simulink model "MHILSimHWImpl"  (R2024a)
settings: Solver=FixedStepDiscrete  StartTime=0.0  StopTime=2e-4  FixedStep=4e-9  RelTol=1e-3
values from neighbouring files (symbols this model uses):
  cfg = tddbl_model    [HILSimModel.m]
undefined symbols (not defined in the file or in its folder): AXI4, dt, hw, ip, Lite, xc7z020clg400
libraries: hdlBasic x1497, hdlUtilities x3, vmcUtilities x1
(part 8 of 11)

== system MHILSimHWImpl/hilsim_ipcore/proc_domain/slice_1/int_xddot_xdot ==
  ts_sync_in : Inport
  reset_in : Inport  Port=2
  xdot : Inport  Port=3
  Constant : hdlBasic/Constant  const=ip.int_dt_residual  gui_display_data_type=Fixed-point  arith_type=Signed (2's comp)  n_bits=dt.const.sz  bin_pt=dt.const.bin  preci_type=Single  exp_width=8  frac_width=24  explicit_period=off  period=1  XmcBlockStatus=1  maskContainerNames=tabcontainer1  block_type=constant  block_config=sysgen:Constant_config
  Register : hdlBasic/Register  init=0  rst=on  en=on  XmcBlockStatus=1  maskContainerNames=tabcontainer1  block_type=register  block_config=sysgen:Register_config
  Register1 : hdlBasic/Register  init=0  rst=on  en=on  XmcBlockStatus=1  maskContainerNames=tabcontainer1  block_type=register  block_config=sysgen:Register_config
  add_stage_1 : hdlBasic/AddSub  mode=Addition  use_carryin=off  use_carryout=off  en=off  latency=1  precision=User Defined  arith_type="Signed  (2's comp)"  n_bits=dt.slice.sz  bin_pt=dt.slice.bin  quantization=Truncate  overflow=Wrap  use_behavioral_HDL=off  hw_selection=Fabric  pipelined=off  XmcBlockStatus=1  maskContainerNames=tabcontainer1  block_type=addsub  block_config=sysgen:Addsub_config
  add_stage_2 : hdlBasic/AddSub  mode=Subtraction  use_carryin=off  use_carryout=off  en=off  latency=1  precision=User Defined  arith_type="Signed  (2's comp)"  n_bits=dt.slice.sz  bin_pt=dt.slice.bin  quantization=Truncate  overflow=Wrap  use_behavioral_HDL=off  hw_selection=Fabric  pipelined=off  XmcBlockStatus=1  maskContainerNames=tabcontainer1  block_type=addsub  block_config=sysgen:Addsub_config
  deltat_residual_mult : hdlBasic/Mult  precision=User Defined  arith_type="Signed  (2's comp)"  n_bits=dt.slice.sz  bin_pt=dt.slice.bin  quantization=Truncate  overflow=Wrap  en=off  latency=2  opt_float=off  fp_mult_usage=No Usage  use_behavioral_HDL=off  opt=Speed  use_embedded=on  optimum_pipeline=off  pipeline=on  use_rpm=on  placement_style=Triangular  XmcBlockStatus=1  maskContainerNames=group1  block_type=mult  block_config=sysgen:Mult_config  block_width=598  block_height=876
  half : hdlBasic/Scale  scale_factor=-1  XmcBlockStatus=1  maskContainerNames=group1  block_type=scale  block_config=sysgen:Scale_config
  int_accum : hdlBasic/AddSub  mode=Addition  use_carryin=off  use_carryout=off  en=off  latency=2  precision=User Defined  arith_type="Signed  (2's comp)"  n_bits=dt.accum.sz  bin_pt=dt.accum.bin  quantization=Truncate  overflow=Saturate  use_behavioral_HDL=off  hw_selection=DSP48  pipelined=on  XmcBlockStatus=1  maskContainerNames=tabcontainer1  block_type=addsub  block_config=sysgen:Addsub_config
  prepend_zeros : hdlBasic/Convert  gui_display_data_type=Fixed-point  arith_type=Signed (2's comp)  n_bits=dt.slice.sz + ip.int_scale_bits  bin_pt=dt.slice.bin  float_type=Single  exp_bits=8  fraction_bits=24  quantization=Truncate  overflow=Wrap  en=off  latency=0  pipeline=off  XmcBlockStatus=1  maskContainerNames=group2  block_type=convert  block_config=sysgen:Convert_config  block_width=595  block_height=885
  shift_prescale : hdlBasic/Scale  scale_factor=-ip.int_scale_bits  XmcBlockStatus=1  maskContainerNames=group1  block_type=scale  block_config=sysgen:Scale_config
  x : Outport
  wires:
  shift_prescale/1 -> int_accum/1
  prepend_zeros/1 -> shift_prescale/1
  Constant/1 -> deltat_residual_mult/2
  deltat_residual_mult/1 -> prepend_zeros/1
  ts_sync_in/1 -> Register/3, Register1/3
  int_accum/1 -> x/1, Register/1
  add_stage_1/1 -> add_stage_2/1
  half/1 -> Register1/1, add_stage_1/2
  reset_in/1 -> Register/2, Register1/2
  Register/1 -> int_accum/2
  Register1/1 -> add_stage_2/2
  xdot/1 -> add_stage_1/1, half/1
  add_stage_2/1 -> deltat_residual_mult/1

== system MHILSimHWImpl/hilsim_ipcore/proc_domain/slice_1/int_xdot_x ==
  ts_sync_in : Inport
  reset_in : Inport  Port=2
  xdot : Inport  Port=3
  Constant : hdlBasic/Constant  const=ip.int_dt_residual  gui_display_data_type=Fixed-point  arith_type=Signed (2's comp)  n_bits=dt.const.sz  bin_pt=dt.const.bin  preci_type=Single  exp_width=8  frac_width=24  explicit_period=off  period=1  XmcBlockStatus=1  maskContainerNames=tabcontainer1  block_type=constant  block_config=sysgen:Constant_config
  Register : hdlBasic/Register  init=0  rst=on  en=on  XmcBlockStatus=1  maskContainerNames=tabcontainer1  block_type=register  block_config=sysgen:Register_config
  Register1 : hdlBasic/Register  init=0  rst=on  en=on  XmcBlockStatus=1  maskContainerNames=tabcontainer1  block_type=register  block_config=sysgen:Register_config
  add_stage_3 : hdlBasic/AddSub  mode=Addition  use_carryin=off  use_carryout=off  en=off  latency=1  precision=User Defined  arith_type="Signed  (2's comp)"  n_bits=dt.slice.sz  bin_pt=dt.slice.bin  quantization=Truncate  overflow=Wrap  use_behavioral_HDL=off  hw_selection=Fabric  pipelined=off  XmcBlockStatus=1  maskContainerNames=tabcontainer1  block_type=addsub  block_config=sysgen:Addsub_config
  deltat_residual_mult : hdlBasic/Mult  precision=User Defined  arith_type="Signed  (2's comp)"  n_bits=dt.slice.sz  bin_pt=dt.slice.bin  quantization=Truncate  overflow=Wrap  en=off  latency=2  opt_float=off  fp_mult_usage=No Usage  use_behavioral_HDL=off  opt=Speed  use_embedded=on  optimum_pipeline=off  pipeline=on  use_rpm=on  placement_style=Triangular  XmcBlockStatus=1  maskContainerNames=group1  block_type=mult  block_config=sysgen:Mult_config  block_width=598  block_height=876
  half1 : hdlBasic/Scale  scale_factor=-1  XmcBlockStatus=1  maskContainerNames=group1  block_type=scale  block_config=sysgen:Scale_config
  int_accum : hdlBasic/AddSub  mode=Addition  use_carryin=off  use_carryout=off  en=off  latency=2  precision=User Defined  arith_type="Signed  (2's comp)"  n_bits=dt.accum.sz  bin_pt=dt.accum.bin  quantization=Truncate  overflow=Saturate  use_behavioral_HDL=off  hw_selection=DSP48  pipelined=on  XmcBlockStatus=1  maskContainerNames=tabcontainer1  block_type=addsub  block_config=sysgen:Addsub_config
  prepend_zeros : hdlBasic/Convert  gui_display_data_type=Fixed-point  arith_type="Signed  (2's comp)"  n_bits=dt.slice.sz + ip.int_scale_bits  bin_pt=dt.slice.bin  float_type=Single  exp_bits=8  fraction_bits=24  quantization=Truncate  overflow=Wrap  en=off  latency=0  pipeline=off  XmcBlockStatus=1  maskContainerNames=group2  block_type=convert  block_config=sysgen:Convert_config  block_width=595  block_height=885
  shift_prescale : hdlBasic/Scale  scale_factor=-ip.int_scale_bits  XmcBlockStatus=1  maskContainerNames=group1  block_type=scale  block_config=sysgen:Scale_config
  x : Outport
  wires:
  shift_prescale/1 -> int_accum/1
  prepend_zeros/1 -> shift_prescale/1
  Constant/1 -> deltat_residual_mult/2
  deltat_residual_mult/1 -> prepend_zeros/1
  int_accum/1 -> Register/1, x/1
  Register/1 -> int_accum/2
  add_stage_3/1 -> half1/1
  Register1/1 -> add_stage_3/2
  ts_sync_in/1 -> Register1/3, Register/3
  reset_in/1 -> Register1/2, Register/2
  xdot/1 -> Register1/1, add_stage_3/1
  half1/1 -> deltat_residual_mult/1

== system MHILSimHWImpl/hilsim_ipcore/proc_domain/slice_1/x_psc ==
  in : Inport
  presc_shift : Inport  Port=2
  presc_mul : Inport  Port=3
  barrel_left_shifter : Subsystem
  cast_to_dt/slice : hdlBasic/Convert  gui_display_data_type=Fixed-point  arith_type="Signed  (2's comp)"  n_bits=dt.slice.sz  bin_pt=dt.slice.bin  float_type=Single  exp_bits=8  fraction_bits=24  quantization=Truncate  overflow=Wrap  en=off  latency=0  pipeline=off  XmcBlockStatus=1  maskContainerNames=group2  block_type=convert  block_config=sysgen:Convert_config  block_width=595  block_height=885
  mult_presc : hdlBasic/Mult  precision=User Defined  arith_type="Signed  (2's comp)"  n_bits=dt.slice.sz  bin_pt=dt.slice.bin  quantization=Truncate  overflow=Wrap  en=off  latency=2  opt_float=off  fp_mult_usage=No Usage  use_behavioral_HDL=off  opt=Speed  use_embedded=on  optimum_pipeline=off  pipeline=on  use_rpm=on  placement_style=Triangular  XmcBlockStatus=1  maskContainerNames=group1  block_type=mult  block_config=sysgen:Mult_config  block_width=598  block_height=876
  out : Outport
  wires:
  presc_mul/1 -> mult_presc/2
  barrel_left_shifter/1(out) -> cast_to_dt/slice/1
  cast_to_dt/slice/1 -> mult_presc/1
  mult_presc/1 -> out/1
  presc_shift/1 -> barrel_left_shifter/2(shift_by)
  in/1 -> barrel_left_shifter/1(in)

== system MHILSimHWImpl/hilsim_ipcore/proc_domain/slice_1/xdot_psc ==
  in : Inport
  presc_shift : Inport  Port=2
  presc_mul : Inport  Port=3
  barrel_left_shifter : Subsystem
  cast_to_dt/slice : hdlBasic/Convert  gui_display_data_type=Fixed-point  arith_type=Signed (2's comp)  n_bits=dt.slice.sz  bin_pt=dt.slice.bin  float_type=Single  exp_bits=8  fraction_bits=24  quantization=Truncate  overflow=Wrap  en=off  latency=0  pipeline=off  XmcBlockStatus=1  maskContainerNames=group2  block_type=convert  block_config=sysgen:Convert_config  block_width=595  block_height=885
  mult_presc : hdlBasic/Mult  precision=User Defined  arith_type="Signed  (2's comp)"  n_bits=dt.slice.sz  bin_pt=dt.slice.bin  quantization=Truncate  overflow=Wrap  en=off  latency=2  opt_float=off  fp_mult_usage=No Usage  use_behavioral_HDL=off  opt=Speed  use_embedded=on  optimum_pipeline=off  pipeline=on  use_rpm=on  placement_style=Triangular  XmcBlockStatus=1  maskContainerNames=group1  block_type=mult  block_config=sysgen:Mult_config  block_width=598  block_height=876
  out : Outport
  wires:
  presc_mul/1 -> mult_presc/2
  barrel_left_shifter/1(out) -> cast_to_dt/slice/1
  cast_to_dt/slice/1 -> mult_presc/1
  mult_presc/1 -> out/1
  presc_shift/1 -> barrel_left_shifter/2(shift_by)
  in/1 -> barrel_left_shifter/1(in)

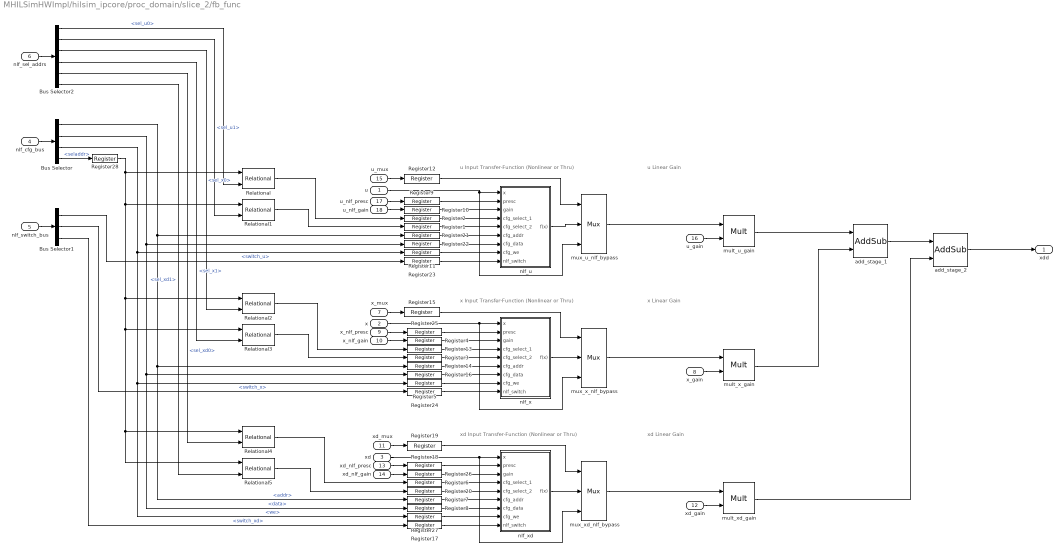
== system MHILSimHWImpl/hilsim_ipcore/proc_domain/slice_2/fb_func ==
  note: u Linear Gain
  note: x Linear Gain
  note: xd Linear Gain
  note: x Input Transfer-Function (Nonlinear or Thru)
  note: xd Input Transfer-Function (Nonlinear or Thru)
  note: u Input Transfer-Function (Nonlinear or Thru)
  u : Inport
  x : Inport  Port=2
  xd : Inport  Port=3
  nlf_cfg_bus : Inport  Port=4
  nlf_switch_bus : Inport  Port=5
  nlf_sel_addrs : Inport  Port=6
  x_mux : Inport  Port=7
  x_gain : Inport  Port=8
  x_nlf_presc : Inport  Port=9
  x_nlf_gain : Inport  Port=10
  xd_mux : Inport  Port=11
  xd_gain : Inport  Port=12
  xd_nlf_presc : Inport  Port=13
  xd_nlf_gain : Inport  Port=14
  u_mux : Inport  Port=15
  u_gain : Inport  Port=16
  u_nlf_presc : Inport  Port=17
  u_nlf_gain : Inport  Port=18
  Bus Selector : BusSelector  OutputSignals=addr,data,we,seladdr
  Bus Selector1 : BusSelector  OutputSignals=switch_u,switch_x,switch_xd
  Bus Selector2 : BusSelector  OutputSignals=sel_u0,sel_u1,sel_x0,sel_x1,sel_xd0,sel_xd1
  Register{1..28} (28 alike) : hdlBasic/Register  init=0  rst=off  en=off  XmcBlockStatus=1  maskContainerNames=tabcontainer1  block_type=register  block_config=sysgen:Register_config
  Relational{,1..5} (6 alike) : hdlBasic/Relational  mode=a=b  op_type=Bool  en=off  latency=1  XmcBlockStatus=1  maskContainerNames=tabcontainer1  block_type=relational  block_config=sysgen:Relational_config
  add_stage_1 : hdlBasic/AddSub  mode=Addition  use_carryin=off  use_carryout=off  en=off  latency=1  precision=User Defined  arith_type="Signed  (2's comp)"  n_bits=dt.slice.sz  bin_pt=dt.slice.bin  quantization=Truncate  overflow=Wrap  use_behavioral_HDL=off  hw_selection=Fabric  pipelined=off  XmcBlockStatus=1  maskContainerNames=tabcontainer1  block_type=addsub  block_config=sysgen:Addsub_config
  add_stage_2 : hdlBasic/AddSub  mode=Addition  use_carryin=off  use_carryout=off  en=off  latency=1  precision=User Defined  arith_type="Signed  (2's comp)"  n_bits=dt.slice.sz  bin_pt=dt.slice.bin  quantization=Truncate  overflow=Wrap  use_behavioral_HDL=off  hw_selection=Fabric  pipelined=off  XmcBlockStatus=1  maskContainerNames=tabcontainer1  block_type=addsub  block_config=sysgen:Addsub_config
  mult_u_gain : hdlBasic/Mult  precision=User Defined  arith_type="Signed  (2's comp)"  n_bits=dt.slice.sz  bin_pt=dt.slice.bin  quantization=Truncate  overflow=Wrap  en=off  latency=2  opt_float=off  fp_mult_usage=No Usage  use_behavioral_HDL=off  opt=Speed  use_embedded=on  optimum_pipeline=off  pipeline=on  use_rpm=on  placement_style=Triangular  XmcBlockStatus=1  maskContainerNames=group1  block_type=mult  block_config=sysgen:Mult_config  block_width=598  block_height=876
  mult_x_gain : hdlBasic/Mult  precision=User Defined  arith_type="Signed  (2's comp)"  n_bits=dt.slice.sz  bin_pt=dt.slice.bin  quantization=Truncate  overflow=Wrap  en=off  latency=2  opt_float=off  fp_mult_usage=No Usage  use_behavioral_HDL=off  opt=Speed  use_embedded=on  optimum_pipeline=off  pipeline=on  use_rpm=on  placement_style=Triangular  XmcBlockStatus=1  maskContainerNames=group1  block_type=mult  block_config=sysgen:Mult_config  block_width=598  block_height=876
  mult_xd_gain : hdlBasic/Mult  precision=User Defined  arith_type="Signed  (2's comp)"  n_bits=dt.slice.sz  bin_pt=dt.slice.bin  quantization=Truncate  overflow=Wrap  en=off  latency=2  opt_float=off  fp_mult_usage=No Usage  use_behavioral_HDL=off  opt=Speed  use_embedded=on  optimum_pipeline=off  pipeline=on  use_rpm=on  placement_style=Triangular  XmcBlockStatus=1  maskContainerNames=group1  block_type=mult  block_config=sysgen:Mult_config  block_width=598  block_height=876
  mux_u_nlf_bypass : hdlBasic/Mux  inputs=2  en=off  latency=1  precision=Full  arith_type=Unsigned  n_bits=16  bin_pt=14  quantization=Truncate  overflow=Wrap  XmcBlockStatus=1  maskContainerNames=tabcontainer1  block_type=mux  block_config=sysgen:Mux_config
  mux_x_nlf_bypass : hdlBasic/Mux  inputs=2  en=off  latency=1  precision=Full  arith_type=Unsigned  n_bits=16  bin_pt=14  quantization=Truncate  overflow=Wrap  XmcBlockStatus=1  maskContainerNames=tabcontainer1  block_type=mux  block_config=sysgen:Mux_config
  mux_xd_nlf_bypass : hdlBasic/Mux  inputs=2  en=off  latency=1  precision=Full  arith_type=Unsigned  n_bits=16  bin_pt=14  quantization=Truncate  overflow=Wrap  XmcBlockStatus=1  maskContainerNames=tabcontainer1  block_type=mux  block_config=sysgen:Mux_config
  nlf_u : Subsystem
  nlf_x : Subsystem
  nlf_xd : Subsystem
  xdd : Outport
  wires:
  x_gain/1 -> mult_x_gain/2
  mux_x_nlf_bypass/1 -> mult_x_gain/1
  x/1 -> nlf_x/1(x), mux_x_nlf_bypass/3
  x_mux/1 -> Register15/1
  nlf_x/1(f(x)) -> mux_x_nlf_bypass/2
  mult_u_gain/1 -> add_stage_1/1
  mult_x_gain/1 -> add_stage_1/2
  add_stage_1/1 -> add_stage_2/1
  mult_xd_gain/1 -> add_stage_2/2
  add_stage_2/1 -> xdd/1
  xd_mux/1 -> Register19/1
  xd/1 -> nlf_xd/1(x), mux_xd_nlf_bypass/3
  mux_xd_nlf_bypass/1 -> mult_xd_gain/1
  nlf_xd/1(f(x)) -> mux_xd_nlf_bypass/2
  xd_gain/1 -> mult_xd_gain/2
  u_gain/1 -> mult_u_gain/2
  u_mux/1 -> Register12/1
  u_nlf_presc/1 -> Register9/1
  u/1 -> mux_u_nlf_bypass/3, nlf_u/1(x)
  u_nlf_gain/1 -> Register10/1
  mux_u_nlf_bypass/1 -> mult_u_gain/1
  nlf_u/1(f(x)) -> mux_u_nlf_bypass/2
  Register9/1 -> nlf_u/2(presc)
  Register10/1 -> nlf_u/3(gain)
  Register12/1 -> mux_u_nlf_bypass/1
  Register15/1 -> mux_x_nlf_bypass/1
  Register19/1 -> mux_xd_nlf_bypass/1
  Register2/1 -> nlf_u/4(cfg_select_1)
  Register1/1 -> nlf_u/5(cfg_select_2)
  Register21/1 -> nlf_u/6(cfg_addr)
  Register22/1 -> nlf_u/7(cfg_data)
  Register11/1 -> nlf_u/8(cfg_we)
  Register23/1 -> nlf_u/9(nlf_switch)
  nlf_cfg_bus/1 -> Bus Selector/1
  Bus Selector/1 -> Register7/1, Register14/1, Register21/1  "<addr>"
  Bus Selector/2 -> Register8/1, Register16/1, Register22/1  "<data>"
  Bus Selector/3 -> Register27/1, Register5/1, Register11/1  "<we>"
  Bus Selector/4 -> Register28/1  "<seladdr>"
  Relational1/1 -> Register1/1
  Relational/1 -> Register2/1
  nlf_switch_bus/1 -> Bus Selector1/1
  Bus Selector1/1 -> Register23/1  "<switch_u>"
  Register5/1 -> nlf_x/8(cfg_we)
  Register16/1 -> nlf_x/7(cfg_data)
  Register14/1 -> nlf_x/6(cfg_addr)
  Register24/1 -> nlf_x/9(nlf_switch)
  Register25/1 -> nlf_x/2(presc)
  Register3/1 -> nlf_x/5(cfg_select_2)
  Register13/1 -> nlf_x/4(cfg_select_1)
  Register4/1 -> nlf_x/3(gain)
  x_nlf_presc/1 -> Register25/1
  x_nlf_gain/1 -> Register4/1
  Relational3/1 -> Register3/1
  Relational2/1 -> Register13/1
  Bus Selector1/2 -> Register24/1  "<switch_x>"
  Register6/1 -> nlf_xd/4(cfg_select_1)
  Register18/1 -> nlf_xd/2(presc)
  Register20/1 -> nlf_xd/5(cfg_select_2)
  Register17/1 -> nlf_xd/9(nlf_switch)
  Register26/1 -> nlf_xd/3(gain)
  Register27/1 -> nlf_xd/8(cfg_we)
  Register8/1 -> nlf_xd/7(cfg_data)
  Register7/1 -> nlf_xd/6(cfg_addr)
  xd_nlf_presc/1 -> Register18/1
  xd_nlf_gain/1 -> Register26/1
  Relational4/1 -> Register6/1
  Relational5/1 -> Register20/1
  Bus Selector1/3 -> Register17/1  "<switch_xd>"
  Register28/1 -> Relational5/1, Relational4/1, Relational3/1, Relational2/1, Relational1/1, Relational/1
  nlf_sel_addrs/1 -> Bus Selector2/1
  Bus Selector2/6 -> Relational5/2  "<sel_xd1>"
  Bus Selector2/5 -> Relational4/2  "<sel_xd0>"
  Bus Selector2/4 -> Relational3/2  "<sel_x1>"
  Bus Selector2/3 -> Relational2/2  "<sel_x0>"
  Bus Selector2/2 -> Relational1/2  "<sel_u1>"
  Bus Selector2/1 -> Relational/2  "<sel_u0>"

== system MHILSimHWImpl/hilsim_ipcore/proc_domain/slice_2/fb_resync ==
  ts_sync_in : Inport
  reset_in : Inport  Port=2
  u : Inport  Port=3
  x : Inport  Port=4
  xd : Inport  Port=5
  xdd : Inport  Port=6
  sync_u : hdlBasic/Register  init=0  rst=on  en=on  XmcBlockStatus=1  maskContainerNames=tabcontainer1  block_type=register  block_config=sysgen:Register_config
  sync_x : hdlBasic/Register  init=0  rst=on  en=on  XmcBlockStatus=1  maskContainerNames=tabcontainer1  block_type=register  block_config=sysgen:Register_config
  sync_xdot : hdlBasic/Register  init=0  rst=on  en=on  XmcBlockStatus=1  maskContainerNames=tabcontainer1  block_type=register  block_config=sysgen:Register_config
  sync_xdotdot : hdlBasic/Register  init=0  rst=on  en=on  XmcBlockStatus=1  maskContainerNames=tabcontainer1  block_type=register  block_config=sysgen:Register_config
  u_sync : Outport
  x_sync : Outport  Port=2
  xd_sync : Outport  Port=3
  xdd_sync : Outport  Port=4
  wires:
  ts_sync_in/1 -> sync_xdotdot/3, sync_xdot/3, sync_x/3, sync_u/3
  u/1 -> sync_u/1
  sync_u/1 -> u_sync/1
  reset_in/1 -> sync_xdot/2, sync_xdotdot/2, sync_x/2, sync_u/2
  sync_x/1 -> x_sync/1
  x/1 -> sync_x/1
  xd/1 -> sync_xdot/1
  sync_xdot/1 -> xd_sync/1
  xdd/1 -> sync_xdotdot/1
  sync_xdotdot/1 -> xdd_sync/1

== system MHILSimHWImpl/hilsim_ipcore/proc_domain/slice_2/int_xddot_xdot ==
  ts_sync_in : Inport
  reset_in : Inport  Port=2
  xdot : Inport  Port=3
  Constant : hdlBasic/Constant  const=ip.int_dt_residual  gui_display_data_type=Fixed-point  arith_type=Signed (2's comp)  n_bits=dt.const.sz  bin_pt=dt.const.bin  preci_type=Single  exp_width=8  frac_width=24  explicit_period=off  period=1  XmcBlockStatus=1  maskContainerNames=tabcontainer1  block_type=constant  block_config=sysgen:Constant_config
  Register : hdlBasic/Register  init=0  rst=on  en=on  XmcBlockStatus=1  maskContainerNames=tabcontainer1  block_type=register  block_config=sysgen:Register_config
  Register1 : hdlBasic/Register  init=0  rst=on  en=on  XmcBlockStatus=1  maskContainerNames=tabcontainer1  block_type=register  block_config=sysgen:Register_config
  add_stage_1 : hdlBasic/AddSub  mode=Addition  use_carryin=off  use_carryout=off  en=off  latency=1  precision=User Defined  arith_type="Signed  (2's comp)"  n_bits=dt.slice.sz  bin_pt=dt.slice.bin  quantization=Truncate  overflow=Wrap  use_behavioral_HDL=off  hw_selection=Fabric  pipelined=off  XmcBlockStatus=1  maskContainerNames=tabcontainer1  block_type=addsub  block_config=sysgen:Addsub_config
  add_stage_2 : hdlBasic/AddSub  mode=Subtraction  use_carryin=off  use_carryout=off  en=off  latency=1  precision=User Defined  arith_type="Signed  (2's comp)"  n_bits=dt.slice.sz  bin_pt=dt.slice.bin  quantization=Truncate  overflow=Wrap  use_behavioral_HDL=off  hw_selection=Fabric  pipelined=off  XmcBlockStatus=1  maskContainerNames=tabcontainer1  block_type=addsub  block_config=sysgen:Addsub_config
  deltat_residual_mult : hdlBasic/Mult  precision=User Defined  arith_type="Signed  (2's comp)"  n_bits=dt.slice.sz  bin_pt=dt.slice.bin  quantization=Truncate  overflow=Wrap  en=off  latency=2  opt_float=off  fp_mult_usage=No Usage  use_behavioral_HDL=off  opt=Speed  use_embedded=on  optimum_pipeline=off  pipeline=on  use_rpm=on  placement_style=Triangular  XmcBlockStatus=1  maskContainerNames=group1  block_type=mult  block_config=sysgen:Mult_config  block_width=598  block_height=876
  half : hdlBasic/Scale  scale_factor=-1  XmcBlockStatus=1  maskContainerNames=group1  block_type=scale  block_config=sysgen:Scale_config
  int_accum : hdlBasic/AddSub  mode=Addition  use_carryin=off  use_carryout=off  en=off  latency=2  precision=User Defined  arith_type="Signed  (2's comp)"  n_bits=dt.accum.sz  bin_pt=dt.accum.bin  quantization=Truncate  overflow=Saturate  use_behavioral_HDL=off  hw_selection=DSP48  pipelined=on  XmcBlockStatus=1  maskContainerNames=tabcontainer1  block_type=addsub  block_config=sysgen:Addsub_config
  prepend_zeros : hdlBasic/Convert  gui_display_data_type=Fixed-point  arith_type="Signed  (2's comp)"  n_bits=dt.slice.sz + ip.int_scale_bits  bin_pt=dt.slice.bin  float_type=Single  exp_bits=8  fraction_bits=24  quantization=Truncate  overflow=Wrap  en=off  latency=0  pipeline=off  XmcBlockStatus=1  maskContainerNames=group2  block_type=convert  block_config=sysgen:Convert_config  block_width=595  block_height=885
  shift_prescale : hdlBasic/Scale  scale_factor=-ip.int_scale_bits  XmcBlockStatus=1  maskContainerNames=group1  block_type=scale  block_config=sysgen:Scale_config
  x : Outport
  wires:
  shift_prescale/1 -> int_accum/1
  prepend_zeros/1 -> shift_prescale/1
  Constant/1 -> deltat_residual_mult/2
  deltat_residual_mult/1 -> prepend_zeros/1
  ts_sync_in/1 -> Register/3, Register1/3
  int_accum/1 -> x/1, Register/1
  add_stage_1/1 -> add_stage_2/1
  half/1 -> Register1/1, add_stage_1/2
  reset_in/1 -> Register/2, Register1/2
  Register/1 -> int_accum/2
  Register1/1 -> add_stage_2/2
  xdot/1 -> add_stage_1/1, half/1
  add_stage_2/1 -> deltat_residual_mult/1

== system MHILSimHWImpl/hilsim_ipcore/proc_domain/slice_2/int_xdot_x ==
  ts_sync_in : Inport
  reset_in : Inport  Port=2
  xdot : Inport  Port=3
  Constant : hdlBasic/Constant  const=ip.int_dt_residual  gui_display_data_type=Fixed-point  arith_type=Signed (2's comp)  n_bits=dt.const.sz  bin_pt=dt.const.bin  preci_type=Single  exp_width=8  frac_width=24  explicit_period=off  period=1  XmcBlockStatus=1  maskContainerNames=tabcontainer1  block_type=constant  block_config=sysgen:Constant_config
  Register : hdlBasic/Register  init=0  rst=on  en=on  XmcBlockStatus=1  maskContainerNames=tabcontainer1  block_type=register  block_config=sysgen:Register_config
  Register1 : hdlBasic/Register  init=0  rst=on  en=on  XmcBlockStatus=1  maskContainerNames=tabcontainer1  block_type=register  block_config=sysgen:Register_config
  add_stage_3 : hdlBasic/AddSub  mode=Addition  use_carryin=off  use_carryout=off  en=off  latency=1  precision=User Defined  arith_type="Signed  (2's comp)"  n_bits=dt.slice.sz  bin_pt=dt.slice.bin  quantization=Truncate  overflow=Wrap  use_behavioral_HDL=off  hw_selection=Fabric  pipelined=off  XmcBlockStatus=1  maskContainerNames=tabcontainer1  block_type=addsub  block_config=sysgen:Addsub_config
  deltat_residual_mult : hdlBasic/Mult  precision=User Defined  arith_type="Signed  (2's comp)"  n_bits=dt.slice.sz  bin_pt=dt.slice.bin  quantization=Truncate  overflow=Wrap  en=off  latency=2  opt_float=off  fp_mult_usage=No Usage  use_behavioral_HDL=off  opt=Speed  use_embedded=on  optimum_pipeline=off  pipeline=on  use_rpm=on  placement_style=Triangular  XmcBlockStatus=1  maskContainerNames=group1  block_type=mult  block_config=sysgen:Mult_config  block_width=598  block_height=876
  half1 : hdlBasic/Scale  scale_factor=-1  XmcBlockStatus=1  maskContainerNames=group1  block_type=scale  block_config=sysgen:Scale_config
  int_accum : hdlBasic/AddSub  mode=Addition  use_carryin=off  use_carryout=off  en=off  latency=2  precision=User Defined  arith_type="Signed  (2's comp)"  n_bits=dt.accum.sz  bin_pt=dt.accum.bin  quantization=Truncate  overflow=Saturate  use_behavioral_HDL=off  hw_selection=DSP48  pipelined=on  XmcBlockStatus=1  maskContainerNames=tabcontainer1  block_type=addsub  block_config=sysgen:Addsub_config
  prepend_zeros : hdlBasic/Convert  gui_display_data_type=Fixed-point  arith_type="Signed  (2's comp)"  n_bits=dt.slice.sz + ip.int_scale_bits  bin_pt=dt.slice.bin  float_type=Single  exp_bits=8  fraction_bits=24  quantization=Truncate  overflow=Wrap  en=off  latency=0  pipeline=off  XmcBlockStatus=1  maskContainerNames=group2  block_type=convert  block_config=sysgen:Convert_config  block_width=595  block_height=885
  shift_prescale : hdlBasic/Scale  scale_factor=-ip.int_scale_bits  XmcBlockStatus=1  maskContainerNames=group1  block_type=scale  block_config=sysgen:Scale_config
  x : Outport
  wires:
  shift_prescale/1 -> int_accum/1
  prepend_zeros/1 -> shift_prescale/1
  Constant/1 -> deltat_residual_mult/2
  deltat_residual_mult/1 -> prepend_zeros/1
  int_accum/1 -> Register/1, x/1
  Register/1 -> int_accum/2
  add_stage_3/1 -> half1/1
  Register1/1 -> add_stage_3/2
  ts_sync_in/1 -> Register1/3, Register/3
  reset_in/1 -> Register1/2, Register/2
  xdot/1 -> Register1/1, add_stage_3/1
  half1/1 -> deltat_residual_mult/1

== system MHILSimHWImpl/hilsim_ipcore/proc_domain/slice_2/x_psc ==
  in : Inport
  presc_shift : Inport  Port=2
  presc_mul : Inport  Port=3
  barrel_left_shifter : Subsystem
  cast_to_dt/slice : hdlBasic/Convert  gui_display_data_type=Fixed-point  arith_type="Signed  (2's comp)"  n_bits=dt.slice.sz  bin_pt=dt.slice.bin  float_type=Single  exp_bits=8  fraction_bits=24  quantization=Truncate  overflow=Wrap  en=off  latency=0  pipeline=off  XmcBlockStatus=1  maskContainerNames=group2  block_type=convert  block_config=sysgen:Convert_config  block_width=595  block_height=885
  mult_presc : hdlBasic/Mult  precision=User Defined  arith_type="Signed  (2's comp)"  n_bits=dt.slice.sz  bin_pt=dt.slice.bin  quantization=Truncate  overflow=Wrap  en=off  latency=2  opt_float=off  fp_mult_usage=No Usage  use_behavioral_HDL=off  opt=Speed  use_embedded=on  optimum_pipeline=off  pipeline=on  use_rpm=on  placement_style=Triangular  XmcBlockStatus=1  maskContainerNames=group1  block_type=mult  block_config=sysgen:Mult_config  block_width=598  block_height=876
  out : Outport
  wires:
  presc_mul/1 -> mult_presc/2
  barrel_left_shifter/1(out) -> cast_to_dt/slice/1
  cast_to_dt/slice/1 -> mult_presc/1
  mult_presc/1 -> out/1
  presc_shift/1 -> barrel_left_shifter/2(shift_by)
  in/1 -> barrel_left_shifter/1(in)

== system MHILSimHWImpl/hilsim_ipcore/proc_domain/slice_2/xdot_psc ==
  in : Inport
  presc_shift : Inport  Port=2
  presc_mul : Inport  Port=3
  barrel_left_shifter : Subsystem
  cast_to_dt/slice : hdlBasic/Convert  gui_display_data_type=Fixed-point  arith_type="Signed  (2's comp)"  n_bits=dt.slice.sz  bin_pt=dt.slice.bin  float_type=Single  exp_bits=8  fraction_bits=24  quantization=Truncate  overflow=Wrap  en=off  latency=0  pipeline=off  XmcBlockStatus=1  maskContainerNames=group2  block_type=convert  block_config=sysgen:Convert_config  block_width=595  block_height=885
  mult_presc : hdlBasic/Mult  precision=User Defined  arith_type="Signed  (2's comp)"  n_bits=dt.slice.sz  bin_pt=dt.slice.bin  quantization=Truncate  overflow=Wrap  en=off  latency=2  opt_float=off  fp_mult_usage=No Usage  use_behavioral_HDL=off  opt=Speed  use_embedded=on  optimum_pipeline=off  pipeline=on  use_rpm=on  placement_style=Triangular  XmcBlockStatus=1  maskContainerNames=group1  block_type=mult  block_config=sysgen:Mult_config  block_width=598  block_height=876
  out : Outport
  wires:
  presc_mul/1 -> mult_presc/2
  barrel_left_shifter/1(out) -> cast_to_dt/slice/1
  cast_to_dt/slice/1 -> mult_presc/1
  mult_presc/1 -> out/1
  presc_shift/1 -> barrel_left_shifter/2(shift_by)
  in/1 -> barrel_left_shifter/1(in)

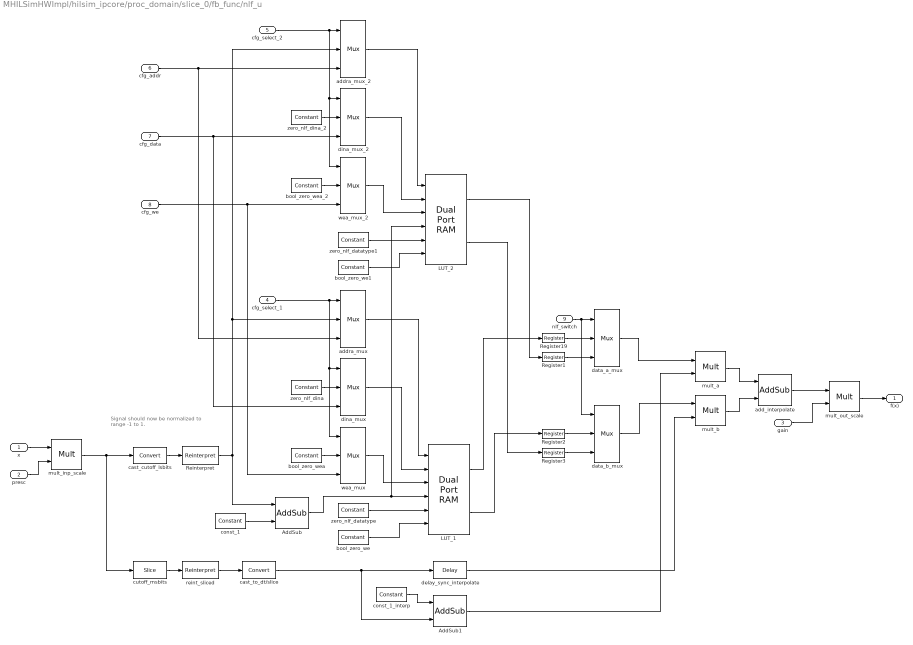
== system MHILSimHWImpl/hilsim_ipcore/proc_domain/slice_0/fb_func/nlf_u ==
  note: Signal should now be normalized
      | to range -1 to 1.
  x : Inport
  presc : Inport  Port=2
  gain : Inport  Port=3
  cfg_select_1 : Inport  Port=4
  cfg_select_2 : Inport  Port=5
  cfg_addr : Inport  Port=6
  cfg_data : Inport  Port=7
  cfg_we : Inport  Port=8
  nlf_switch : Inport  Port=9
  AddSub : hdlBasic/AddSub  mode=Addition  use_carryin=off  use_carryout=off  en=off  latency=1  precision=User Defined  arith_type=Unsigned  n_bits=ip.f_nlf.lut_addr_bits  bin_pt=0  quantization=Truncate  overflow=Wrap  use_behavioral_HDL=off  hw_selection=Fabric  pipelined=off  XmcBlockStatus=1  maskContainerNames=tabcontainer1  block_type=addsub  block_config=sysgen:Addsub_config
  AddSub1 : hdlBasic/AddSub  mode=Subtraction  use_carryin=off  use_carryout=off  en=off  latency=4  precision=User Defined  arith_type="Signed  (2's comp)"  n_bits=dt.slice.sz  bin_pt=dt.slice.bin  quantization=Truncate  overflow=Wrap  use_behavioral_HDL=off  hw_selection=Fabric  pipelined=off  XmcBlockStatus=1  maskContainerNames=tabcontainer1  block_type=addsub  block_config=sysgen:Addsub_config
  LUT_1 : hdlBasic/Dual Port RAM  depth=ip.f_nlf.lut_sz  initVector=cfg.slice0.u_nlf.lut  distributed_mem=Block RAM  init_a=0  init_b=0  rst_a=off  rst_b=off  en_a=off  en_b=off  latency=1  write_mode_A=Read After Write  write_mode_B=Read After Write  explicit_period=[]  period=[]  simulation_type=fast_sim  XmcBlockStatus=1  maskContainerNames=tabcontainer1  block_type=dpram  block_config=sysgen:Dpram_config  optimize=Area
      settings: infoedit=[]
  LUT_2 : hdlBasic/Dual Port RAM  depth=ip.f_nlf.lut_sz  initVector=cfg.slice0.u_nlf.lut  distributed_mem=Block RAM  init_a=0  init_b=0  rst_a=off  rst_b=off  en_a=off  en_b=off  latency=1  write_mode_A=Read After Write  write_mode_B=Read After Write  explicit_period=[]  period=[]  simulation_type=fast_sim  XmcBlockStatus=1  maskContainerNames=tabcontainer1  block_type=dpram  block_config=sysgen:Dpram_config  optimize=Area
      settings: infoedit=[]
  Register{1..3,19} (4 alike) : hdlBasic/Register  init=0  rst=off  en=off  XmcBlockStatus=1  maskContainerNames=tabcontainer1  block_type=register  block_config=sysgen:Register_config
  Reinterpret : hdlBasic/Reinterpret  force_arith_type=on  arith_type=Unsigned  force_bin_pt=on  bin_pt=0  XmcBlockStatus=1  maskContainerNames=group1  block_type=reinterpret  block_config=sysgen:Reinterpret_config
  add_interpolate : hdlBasic/AddSub  mode=Addition  use_carryin=off  use_carryout=off  en=off  latency=1  precision=User Defined  arith_type="Signed  (2's comp)"  n_bits=dt.slice.sz  bin_pt=dt.slice.bin  quantization=Truncate  overflow=Wrap  use_behavioral_HDL=off  hw_selection=Fabric  pipelined=off  XmcBlockStatus=1  maskContainerNames=tabcontainer1  block_type=addsub  block_config=sysgen:Addsub_config
  addra_mux : hdlBasic/Mux  inputs=2  en=off  latency=1  precision=Full  arith_type=Unsigned  n_bits=16  bin_pt=14  quantization=Truncate  overflow=Wrap  XmcBlockStatus=1  maskContainerNames=tabcontainer1  block_type=mux  block_config=sysgen:Mux_config
  "addra_mux_2 " : hdlBasic/Mux  inputs=2  en=off  latency=1  precision=Full  arith_type=Unsigned  n_bits=16  bin_pt=14  quantization=Truncate  overflow=Wrap  XmcBlockStatus=1  maskContainerNames=tabcontainer1  block_type=mux  block_config=sysgen:Mux_config
  bool_zero_we : hdlBasic/Constant  const=0  gui_display_data_type=Boolean  arith_type=Boolean  n_bits=16  bin_pt=14  preci_type=Single  exp_width=8  frac_width=24  explicit_period=off  period=1  XmcBlockStatus=1  maskContainerNames=tabcontainer1  block_type=constant  block_config=sysgen:Constant_config
  bool_zero_we1 : hdlBasic/Constant  const=0  gui_display_data_type=Boolean  arith_type=Boolean  n_bits=16  bin_pt=14  preci_type=Single  exp_width=8  frac_width=24  explicit_period=off  period=1  XmcBlockStatus=1  maskContainerNames=tabcontainer1  block_type=constant  block_config=sysgen:Constant_config
  bool_zero_wea : hdlBasic/Constant  const=0  gui_display_data_type=Boolean  arith_type=Boolean  n_bits=16  bin_pt=14  preci_type=Single  exp_width=8  frac_width=24  explicit_period=off  period=1  XmcBlockStatus=1  maskContainerNames=tabcontainer1  block_type=constant  block_config=sysgen:Constant_config
  bool_zero_wea_2 : hdlBasic/Constant  const=0  gui_display_data_type=Boolean  arith_type=Boolean  n_bits=16  bin_pt=14  preci_type=Single  exp_width=8  frac_width=24  explicit_period=off  period=1  XmcBlockStatus=1  maskContainerNames=tabcontainer1  block_type=constant  block_config=sysgen:Constant_config
  cast_cutoff_lsbits : hdlBasic/Convert  gui_display_data_type=Fixed-point  arith_type="Signed  (2's comp)"  n_bits=ip.f_nlf.lut_addr_bits  bin_pt=ip.f_nlf.lut_addr_bits-1  float_type=Single  exp_bits=8  fraction_bits=24  quantization=Truncate  overflow=Wrap  en=off  latency=0  pipeline=off  XmcBlockStatus=1  maskContainerNames=group2  block_type=convert  block_config=sysgen:Convert_config  block_width=595  block_height=885
  cast_to_dt/slice : hdlBasic/Convert  gui_display_data_type=Fixed-point  arith_type="Signed  (2's comp)"  n_bits=dt.slice.sz  bin_pt=dt.slice.bin  float_type=Single  exp_bits=8  fraction_bits=24  quantization=Truncate  overflow=Wrap  en=off  latency=0  pipeline=off  XmcBlockStatus=1  maskContainerNames=group2  block_type=convert  block_config=sysgen:Convert_config  block_width=595  block_height=885
  const_1 : hdlBasic/Constant  const=1.0  gui_display_data_type=Fixed-point  arith_type=Unsigned  n_bits=ip.f_nlf.lut_addr_bits  bin_pt=0  preci_type=Single  exp_width=8  frac_width=24  explicit_period=off  period=1  XmcBlockStatus=1  maskContainerNames=tabcontainer1  block_type=constant  block_config=sysgen:Constant_config
  const_1_interp : hdlBasic/Constant  const=1  gui_display_data_type=Fixed-point  arith_type=Signed (2's comp)  n_bits=dt.slice.sz  bin_pt=dt.slice.bin  preci_type=Single  exp_width=8  frac_width=24  explicit_period=off  period=1  XmcBlockStatus=1  maskContainerNames=tabcontainer1  block_type=constant  block_config=sysgen:Constant_config
  cutoff_msbits : hdlBasic/Slice  nbits=dt.slice.sz - ip.f_nlf.lut_addr_bits-1  boolean_output=off  mode=Lower Bit Location + Width  bit1=0  base1=MSB of Input  bit0=0  base0=LSB of Input  XmcBlockStatus=1  maskContainerNames=group1  block_type=slice  block_config=sysgen:Slice_config
  data_a_mux : hdlBasic/Mux  inputs=2  en=off  latency=1  precision=Full  arith_type=Unsigned  n_bits=16  bin_pt=14  quantization=Truncate  overflow=Wrap  XmcBlockStatus=1  maskContainerNames=tabcontainer1  block_type=mux  block_config=sysgen:Mux_config
  data_b_mux : hdlBasic/Mux  inputs=2  en=off  latency=1  precision=Full  arith_type=Unsigned  n_bits=16  bin_pt=14  quantization=Truncate  overflow=Wrap  XmcBlockStatus=1  maskContainerNames=tabcontainer1  block_type=mux  block_config=sysgen:Mux_config
  delay_sync_interpolate : hdlBasic/Delay  rst=off  en=off  latency=4  reg_retiming=off  XmcBlockStatus=1  maskContainerNames=group1  block_type=delay  block_config=sysgen:Delay_config
  dina_mux : hdlBasic/Mux  inputs=2  en=off  latency=1  precision=Full  arith_type=Unsigned  n_bits=16  bin_pt=14  quantization=Truncate  overflow=Wrap  XmcBlockStatus=1  maskContainerNames=tabcontainer1  block_type=mux  block_config=sysgen:Mux_config
  dina_mux_2 : hdlBasic/Mux  inputs=2  en=off  latency=1  precision=Full  arith_type=Unsigned  n_bits=16  bin_pt=14  quantization=Truncate  overflow=Wrap  XmcBlockStatus=1  maskContainerNames=tabcontainer1  block_type=mux  block_config=sysgen:Mux_config
  mult_a : hdlBasic/Mult  precision=User Defined  arith_type="Signed  (2's comp)"  n_bits=dt.slice.sz  bin_pt=dt.slice.bin  quantization=Truncate  overflow=Wrap  en=off  latency=2  opt_float=off  fp_mult_usage=No Usage  use_behavioral_HDL=off  opt=Speed  use_embedded=on  optimum_pipeline=off  pipeline=on  use_rpm=on  placement_style=Triangular  XmcBlockStatus=1  maskContainerNames=group1  block_type=mult  block_config=sysgen:Mult_config  block_width=598  block_height=876
  mult_b : hdlBasic/Mult  precision=User Defined  arith_type="Signed  (2's comp)"  n_bits=dt.slice.sz  bin_pt=dt.slice.bin  quantization=Truncate  overflow=Wrap  en=off  latency=2  opt_float=off  fp_mult_usage=No Usage  use_behavioral_HDL=off  opt=Speed  use_embedded=on  optimum_pipeline=off  pipeline=on  use_rpm=on  placement_style=Triangular  XmcBlockStatus=1  maskContainerNames=group1  block_type=mult  block_config=sysgen:Mult_config  block_width=598  block_height=876
  mult_inp_scale : hdlBasic/Mult  precision=User Defined  arith_type="Signed  (2's comp)"  n_bits=dt.slice.sz  bin_pt=dt.slice.sz - 2  quantization=Truncate  overflow=Wrap  en=off  latency=2  opt_float=off  fp_mult_usage=No Usage  use_behavioral_HDL=off  opt=Speed  use_embedded=on  optimum_pipeline=off  pipeline=on  use_rpm=on  placement_style=Triangular  XmcBlockStatus=1  maskContainerNames=group1  block_type=mult  block_config=sysgen:Mult_config  block_width=598  block_height=876
  mult_out_scale : hdlBasic/Mult  precision=User Defined  arith_type="Signed  (2's comp)"  n_bits=dt.slice.sz  bin_pt=dt.slice.bin  quantization=Truncate  overflow=Wrap  en=off  latency=2  opt_float=off  fp_mult_usage=No Usage  use_behavioral_HDL=off  opt=Speed  use_embedded=on  optimum_pipeline=off  pipeline=on  use_rpm=on  placement_style=Triangular  XmcBlockStatus=1  maskContainerNames=group1  block_type=mult  block_config=sysgen:Mult_config  block_width=598  block_height=876
  reint_sliced : hdlBasic/Reinterpret  force_arith_type=on  arith_type=Unsigned  force_bin_pt=on  bin_pt=dt.slice.sz - ip.f_nlf.lut_addr_bits-1  XmcBlockStatus=1  maskContainerNames=group1  block_type=reinterpret  block_config=sysgen:Reinterpret_config
  wea_mux : hdlBasic/Mux  inputs=2  en=off  latency=1  precision=Full  arith_type=Unsigned  n_bits=16  bin_pt=14  quantization=Truncate  overflow=Wrap  XmcBlockStatus=1  maskContainerNames=tabcontainer1  block_type=mux  block_config=sysgen:Mux_config
  wea_mux_2 : hdlBasic/Mux  inputs=2  en=off  latency=1  precision=Full  arith_type=Unsigned  n_bits=16  bin_pt=14  quantization=Truncate  overflow=Wrap  XmcBlockStatus=1  maskContainerNames=tabcontainer1  block_type=mux  block_config=sysgen:Mux_config
  zero_nlf_datatype : hdlBasic/Constant  const=0  gui_display_data_type=Fixed-point  arith_type=Signed (2's comp)  n_bits=dt.nlf.sz  bin_pt=dt.nlf.bin  preci_type=Single  exp_width=8  frac_width=24  explicit_period=off  period=1  XmcBlockStatus=1  maskContainerNames=tabcontainer1  block_type=constant  block_config=sysgen:Constant_config
  zero_nlf_datatype1 : hdlBasic/Constant  const=0  gui_display_data_type=Fixed-point  arith_type=Signed (2's comp)  n_bits=dt.nlf.sz  bin_pt=dt.nlf.bin  preci_type=Single  exp_width=8  frac_width=24  explicit_period=off  period=1  XmcBlockStatus=1  maskContainerNames=tabcontainer1  block_type=constant  block_config=sysgen:Constant_config
  zero_nlf_dina : hdlBasic/Constant  const=0  gui_display_data_type=Fixed-point  arith_type=Signed (2's comp)  n_bits=dt.nlf.sz  bin_pt=dt.nlf.bin  preci_type=Single  exp_width=8  frac_width=24  explicit_period=off  period=1  XmcBlockStatus=1  maskContainerNames=tabcontainer1  block_type=constant  block_config=sysgen:Constant_config
  zero_nlf_dina_2 : hdlBasic/Constant  const=0  gui_display_data_type=Fixed-point  arith_type=Signed (2's comp)  n_bits=dt.nlf.sz  bin_pt=dt.nlf.bin  preci_type=Single  exp_width=8  frac_width=24  explicit_period=off  period=1  XmcBlockStatus=1  maskContainerNames=tabcontainer1  block_type=constant  block_config=sysgen:Constant_config
  f(x) : Outport
  wires:
  x/1 -> mult_inp_scale/1
  presc/1 -> mult_inp_scale/2
  cast_cutoff_lsbits/1 -> Reinterpret/1
  Reinterpret/1 -> "addra_mux_2 "/2, addra_mux/2, AddSub/1
  const_1/1 -> AddSub/2
  AddSub/1 -> LUT_2/4, LUT_1/4
  bool_zero_we/1 -> LUT_1/6
  zero_nlf_datatype/1 -> LUT_1/5
  mult_inp_scale/1 -> cast_cutoff_lsbits/1, cutoff_msbits/1
  cutoff_msbits/1 -> reint_sliced/1
  reint_sliced/1 -> cast_to_dt/slice/1
  cast_to_dt/slice/1 -> AddSub1/2, delay_sync_interpolate/1
  const_1_interp/1 -> AddSub1/1
  delay_sync_interpolate/1 -> mult_b/2
  AddSub1/1 -> mult_a/2
  mult_a/1 -> add_interpolate/1
  mult_b/1 -> add_interpolate/2
  gain/1 -> mult_out_scale/2
  mult_out_scale/1 -> f(x)/1
  dina_mux/1 -> LUT_1/2
  addra_mux/1 -> LUT_1/1
  wea_mux/1 -> LUT_1/3
  bool_zero_wea/1 -> wea_mux/2
  zero_nlf_dina/1 -> dina_mux/2
  cfg_select_1/1 -> wea_mux/1, dina_mux/1, addra_mux/1
  cfg_addr/1 -> "addra_mux_2 "/3, addra_mux/3
  cfg_we/1 -> wea_mux_2/3, wea_mux/3
  add_interpolate/1 -> mult_out_scale/1
  wea_mux_2/1 -> LUT_2/3
  dina_mux_2/1 -> LUT_2/2
  bool_zero_wea_2/1 -> wea_mux_2/2
  cfg_select_2/1 -> wea_mux_2/1, dina_mux_2/1, "addra_mux_2 "/1
  zero_nlf_dina_2/1 -> dina_mux_2/2
  "addra_mux_2 "/1 -> LUT_2/1
  zero_nlf_datatype1/1 -> LUT_2/5
  bool_zero_we1/1 -> LUT_2/6
  cfg_data/1 -> dina_mux_2/3, dina_mux/3
  LUT_1/1 -> Register19/1
  LUT_2/1 -> Register1/1
  data_a_mux/1 -> mult_a/1
  data_b_mux/1 -> mult_b/1
  LUT_1/2 -> Register2/1
  LUT_2/2 -> Register3/1
  nlf_switch/1 -> data_b_mux/1, data_a_mux/1
  Register19/1 -> data_a_mux/2
  Register1/1 -> data_a_mux/3
  Register2/1 -> data_b_mux/2
  Register3/1 -> data_b_mux/3
